simulink model "Aula7_1_b"  (R2013b)
settings: Solver=ode3  StartTime=0.0  StopTime=10  FixedStep=0.01  RelTol=1e-3
values from neighbouring files (symbols this model uses):
  Ke = (acker(A',C',J)')    [aula7_1_cal_obs.m]
libraries: simulink x2
settings Model: Creator=ThiagoCordeiro  LastModifiedBy=thiag

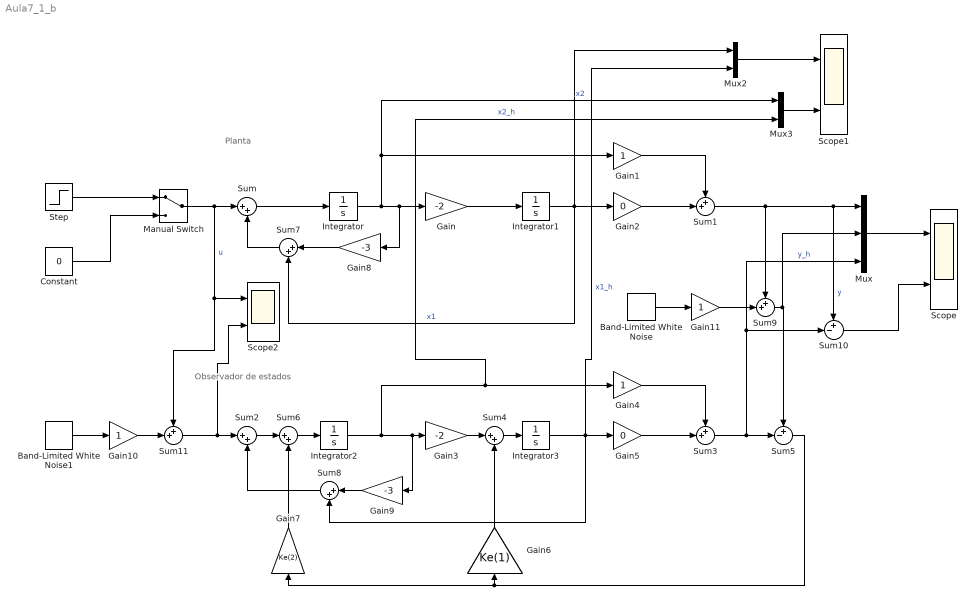
== system Aula7_1_b ==
  note: Planta
  note: Observador de estados
  Band-Limited White Noise : simulink/Sources/Band-Limited White Noise  Cov=[0.01]  Ts=0.01  seed=[23341]
  Band-Limited White Noise1 : simulink/Sources/Band-Limited White Noise  Cov=[0.1]  Ts=0.01  seed=[23341]
  Constant : Constant  Value=0
  Gain : Gain  Gain=-2
  Gain{1,4,10..11} (4 alike) : Gain
  Gain2 : Gain  Gain=0
  Gain3 : Gain  Gain=-2
  Gain5 : Gain  Gain=0
  Gain6 : Gain  Gain=Ke(1)
  Gain7 : Gain  Gain=Ke(2)
  Gain8 : Gain  Gain=-3
  Gain9 : Gain  Gain=-3
  Integrator : Integrator  InitialCondition=10
  Integrator1 : Integrator
  Integrator2 : Integrator
  Integrator3 : Integrator
  Manual Switch : ManualSwitch
  Mux : Mux  Inputs=3
  Mux2 : Mux  Inputs=2
  Mux3 : Mux  Inputs=2
  Scope : Scope  NumInputPorts=2
      settings: YMin=-5~-5  YMax=5~5
  Scope1 : Scope  NumInputPorts=2
      settings: YMin=-5~-5  YMax=5~5
  Scope2 : Scope  NumInputPorts=2
      settings: YMin=-5~-5  YMax=5~5  SaveName=ScopeData2
  Step : Step  Time=0  After=-10  SampleTime=0
  Sum{,2,4,6..8} (6 alike) : Sum  Inputs=|++
  Sum{1,3,9,11} (4 alike) : Sum  Inputs=++|
  Sum10 : Sum  Inputs=+-|
  Sum5 : Sum  Inputs=+-|
  wires:
  Step/1 -> Manual Switch/1
  Sum/1 -> Integrator/1
  Constant/1 -> Manual Switch/2
  Integrator/1 -> Mux3/1, Gain1/1, Gain8/1, Gain/1  "x2"
  Gain/1 -> Integrator1/1
  Integrator1/1 -> Mux2/1, Gain2/1, Sum7/2  "x1"
  Gain2/1 -> Sum1/2
  Gain1/1 -> Sum1/1
  Sum1/1 -> Sum9/1, Sum10/1, Mux/1  "y"
  Manual Switch/1 -> Scope2/1, Sum11/1, Sum/1  "u"
  Integrator2/1 -> Mux3/2, Gain4/1, Gain9/1, Gain3/1  "x2_h"
  Integrator3/1 -> Mux2/2, Sum8/2, Gain5/1  "x1_h"
  Gain5/1 -> Sum3/2
  Gain4/1 -> Sum3/1
  Sum3/1 -> Sum10/2, Mux/3, Sum5/2  "y_h"
  Gain3/1 -> Sum4/1
  Sum4/1 -> Integrator3/1
  Gain6/1 -> Sum4/2
  Sum5/1 -> Gain6/1, Gain7/1
  Sum2/1 -> Sum6/1
  Sum6/1 -> Integrator2/1
  Gain7/1 -> Sum6/2
  Gain8/1 -> Sum7/1
  Sum7/1 -> Sum/2
  Gain9/1 -> Sum8/1
  Sum8/1 -> Sum2/2
  Sum9/1 -> Mux/2, Sum5/1
  Sum10/1 -> Scope/2
  Mux/1 -> Scope/1
  Sum11/1 -> Scope2/2, Sum2/1
  Band-Limited White Noise1/1 -> Gain10/1
  Gain10/1 -> Sum11/2
  Band-Limited White Noise/1 -> Gain11/1
  Gain11/1 -> Sum9/2
  Mux2/1 -> Scope1/1
  Mux3/1 -> Scope1/2
